simulink model "model_simulink"  (R2014b)
settings: Solver=VariableStepAuto  StartTime=0.0  StopTime=30  RelTol=1e-3
libraries: simulink x1
settings Model: Creator=Abdulrhman Tarek  LastModifiedBy=ABDO
settings DataIOCC: LimitDataPoints=off  SaveFormat=Dataset
settings OptimizationCC: UseDivisionForNetSlopeComputation=off  SimCompilerOptimization=off
settings DebuggingCC: SolverPrmCheckMsg=none  FrameProcessingCompatibilityMsg=error
settings HardwareCC: ProdBitPerPointer=64  ProdLargestAtomicFloat=Float  ProdIntDivRoundTo=Zero  ProdEndianess=LittleEndian  ProdWordSize=64  ProdHWDeviceType=Intel->x86-64 (Windows64)
settings ModelReferenceCC: PropagateSignalLabelsOutOfModel=on
settings RTWCC: RTWCompilerOptimization=off
settings ConfigComp: CovMetricSettings=dw  CovHtmlReporting=on  CovSaveCumulativeToWorkspaceVar=on  CovSaveSingleToWorkspaceVar=on  CovExternalEMLEnable=off

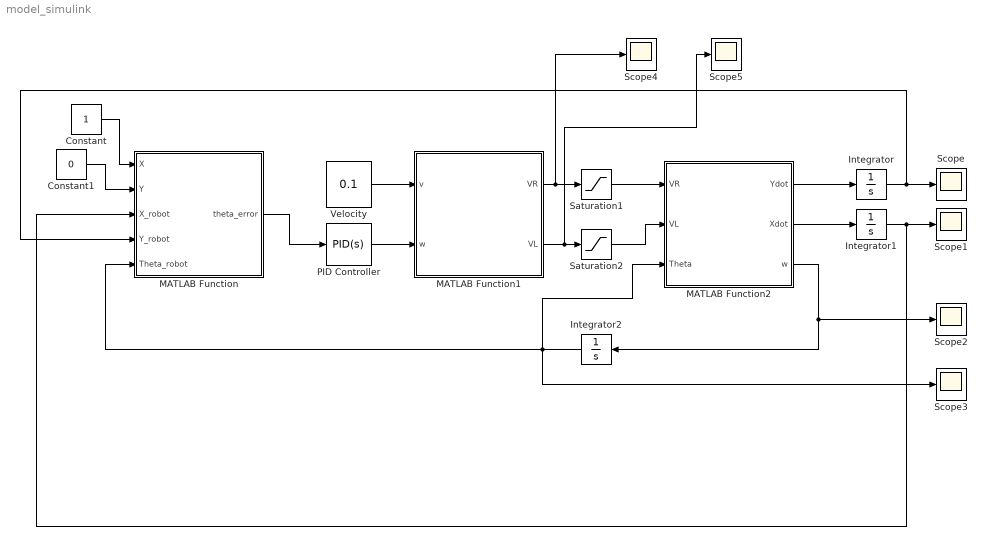
== system model_simulink ==
  Constant : Constant
  Constant1 : Constant  Value=0
  Integrator : Integrator
  Integrator1 : Integrator
  Integrator2 : Integrator
  MATLAB Function : MATLAB Function  TreatAsAtomicUnit=on
  MATLAB Function1 : MATLAB Function  TreatAsAtomicUnit=on
  MATLAB Function2 : MATLAB Function  TreatAsAtomicUnit=on
  PID Controller : simulink/Continuous/PID Controller  Controller=PID  TimeDomain=Continuous-time  SampleTime=-1  IntegratorMethod=Forward Euler  FilterMethod=Forward Euler  Form=Parallel  P=1  I=1  D=0  N=100  InitialConditionSource=internal  InitialConditionForIntegrator=0  InitialConditionForFilter=0  ExternalReset=none  LimitOutput=off  UpperSaturationLimit=inf  LowerSaturationLimit=-inf  LinearizeAsGain=on  AntiWindupMode=none  Kb=1  TrackingMode=off  Kt=1  PParamMin=[]  PParamMax=[]  IParamMin=[]  IParamMax=[]  DParamMin=[]  DParamMax=[]  NParamMin=[]  NParamMax=[]  KbParamMin=[]  KbParamMax=[]  KtParamMin=[]  KtParamMax=[]  POutMin=[]  POutMax=[]  IOutMin=[]  IOutMax=[]  DOutMin=[]  DOutMax=[]  NOutMin=[]  NOutMax=[]  KbOutMin=[]  KbOutMax=[]  KtOutMin=[]  KtOutMax=[]  IntegratorOutMin=[]  IntegratorOutMax=[]  FilterOutMin=[]  FilterOutMax=[]  SumOutMin=[]  SumOutMax=[]  SumI1OutMin=[]  SumI1OutMax=[]  SumI2OutMin=[]  SumI2OutMax=[]  SumI3OutMin=[]  SumI3OutMax=[]  SumDOutMin=[]  SumDOutMax=[]  SaturationOutMin=[]  SaturationOutMax=[]  IntegratorContinuousStateAttributes=''  IntegratorStateMustResolveToSignalObject=off  IntegratorRTWStateStorageClass=Auto  FilterContinuousStateAttributes=''  FilterStateMustResolveToSignalObject=off  FilterRTWStateStorageClass=Auto  DifferentiatorICPrevScaledInput=0  DifferentiatorOutMin=[]  DifferentiatorOutMax=[]  UseFilter=on
  Saturation1 : Saturate  UpperLimit=0.4188  LowerLimit=-0.4188
  Saturation2 : Saturate  UpperLimit=0.4188  LowerLimit=-0.4188
  Scope{,1..5} (6 alike) : Scope
      Scope settings: YMin=-3e-11  YMax=3e-11
      Scope1 settings: YMin=0.2  YMax=2.2
      Scope2 settings: YMin=-0.69714  YMax=6.2819  SaveName=ScopeData2
      Scope3 settings: YMin=-0.39268  YMax=3.53411  SaveName=ScopeData3
      Scope4 settings: YMin=-0.418801  YMax=-0.418792  SaveName=ScopeData4
      Scope5 settings: SaveName=ScopeData5
  "Velocity " : Constant  Value=0.1
  wires:
  MATLAB Function1/2(VL) -> Scope5/1, Saturation2/1
  MATLAB Function1/1(VR) -> Scope4/1, Saturation1/1
  "Velocity "/1 -> MATLAB Function1/1(v)
  PID Controller/1 -> MATLAB Function1/2(w)
  MATLAB Function/1(theta_error) -> PID Controller/1
  Saturation1/1 -> MATLAB Function2/1(VR)
  MATLAB Function2/2(Xdot) -> Integrator1/1
  MATLAB Function2/1(Ydot) -> Integrator/1
  MATLAB Function2/3(w) -> Scope2/1, Integrator2/1
  Integrator1/1 -> MATLAB Function/3(X_robot), Scope1/1
  Saturation2/1 -> MATLAB Function2/2(VL)
  Constant/1 -> MATLAB Function/1(X)
  Constant1/1 -> MATLAB Function/2(Y)
  Integrator/1 -> MATLAB Function/4(Y_robot), Scope/1
  Integrator2/1 -> Scope3/1, MATLAB Function2/3(Theta), MATLAB Function/5(Theta_robot)

== matlab function model_simulink/MATLAB Function1 ==
  data: v input; VR output; w input; VL output
function [VR, VL] = fcn(v, w)
%#codegen
L = 0.15;
R=0.02;
C=1;
VR = v + (w*L)/2 /(C*R);
VL = v - (w*L)/2 /(C*R);

== matlab function model_simulink/MATLAB Function ==
  data: X input; theta_error output; Y input; X_robot input; Y_robot input; Theta_robot input
function theta_error = fcn(X,Y,X_robot,Y_robot,Theta_robot)

theta_error = atan2(Y-Y_robot,X-X_robot)-Theta_robot;

== matlab function model_simulink/MATLAB Function2 ==
  data: VR input; Ydot output; VL input; Xdot output; w output; Theta input
function [Ydot, Xdot, w] = fcn(VR, VL,Theta)
%#codegen
L = 0.15;
v = (VR+VL)/2;
w = (VR-VL)/L
Xdot = v*cos(Theta);
Ydot = v*sin(Theta);
